simulink model "MSD_System"  (R2020a)
settings: Solver=VariableStepAuto  StartTime=0.0  StopTime=10.0  RelTol=1e-3
PostLoadFcn:
  |  b=50;
  | K1=50;
  | M1=100;
  | M2=30;
  | u=5/pi;
libraries: simulink x1
settings Model: DataDictionary=Data.sldd  Creator=NIKITA  LastModifiedBy=NIKITA

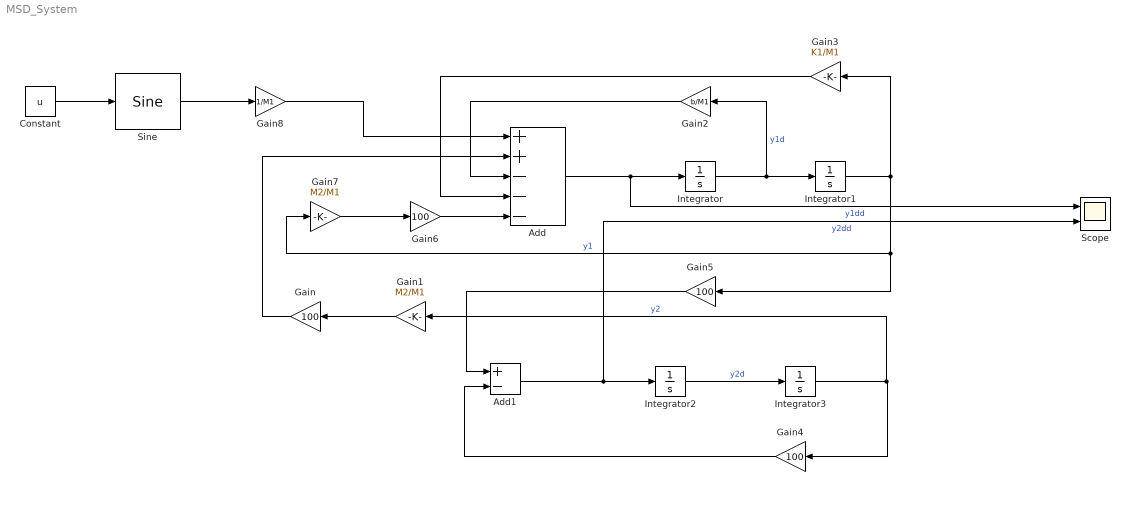
== system MSD_System ==
  Add : Sum  Inputs=++---
  Add1 : Sum  Inputs=+-
  Constant : Constant  Value=u
  Gain{,4..6} (4 alike) : Gain  Gain=100
  Gain1 : Gain  Gain=M2/M1
  Gain2 : Gain  Gain=b/M1
  Gain3 : Gain  Gain=K1/M1
  Gain7 : Gain  Gain=M2/M1
  Gain8 : Gain  Gain=1/M1
  Integrator{,1..3} (4 alike) : Integrator
  Scope : Scope  NumInputPorts=2
  Sine : simulink/Lookup Tables/Sine  Formula=sin(2*pi*u)  NumDataPoints=(2^5)+1  OutputWordLength=16  InternalRulePriority=Speed
  wires:
  Integrator2/1 -> Integrator3/1  "y2d"
  Integrator/1 -> Gain2/1, Integrator1/1  "y1d"
  Add/1 -> Scope/1, Integrator/1  "y1dd"
  Add1/1 -> Scope/2, Integrator2/1  "y2dd"
  Integrator1/1 -> Gain7/1, Gain5/1, Gain3/1  "y1"
  Integrator3/1 -> Gain4/1, Gain1/1  "y2"
  Gain4/1 -> Add1/2
  Gain5/1 -> Add1/1
  Gain/1 -> Add/2
  Gain1/1 -> Gain/1
  Gain7/1 -> Gain6/1
  Gain6/1 -> Add/5
  Sine/1 -> Gain8/1
  Constant/1 -> Sine/1
  Gain8/1 -> Add/1
  Gain3/1 -> Add/4
  Gain2/1 -> Add/3
